simulink model "Template_Simulink_Model_QuanserDCMotor"  (R2018b)
settings: Solver=ode1  StartTime=0.0  StopTime=10  FixedStep=0.001  RelTol=1e-3  EnableMultiTasking=on
undefined symbols (not defined in the file or in its folder): HIL, wf
libraries: quarc_library x3, simulink x1
settings Model: SimulationMode=external  ExtModeTrigDuration=100000  Creator=My Project  LastModifiedBy=Myadmin
settings SolverCC: PositivePriorityOrder=on
settings RTWCC: SystemTargetFile=quarc_linux_rt_armv7.tlc  TemplateMakefile=quarc_linux_rt_armv7_tmf  Description=QUARC Linux RT ARMv7 Target (NI ELVIS III, NI myRIO)
settings STFCustomTargetCC: TargetLibSuffix=.a  TargetPreCompLibLocation=C:\PROGRA~3\QUARC\lib\2018b\LINUX_~1\release  TargetLangStandard=C99 (ISO)  ConcurrentExecutionCompliant=on  GRTInterface=on  SystemTargetFile=quarc_linux_rt_armv7.tlc
settings GRTTargetCC: TargetLibSuffix=.a  TargetPreCompLibLocation=C:\PROGRA~3\QUARC\lib\2018b\LINUX_~1\release  ParMdlRefBuildCompliant=off  CompOptLevelCompliant=off  CombineOutputUpdateFcns=off  MatFileLogging=off  CPPClassGenCompliant=off  GRTInterface=on  UseToolchainInfoCompliant=off  ExtMode=on  ExtModeMexFile=quarc_comm  ExtModeMexArgs='-w -d /tmp -uri %u'

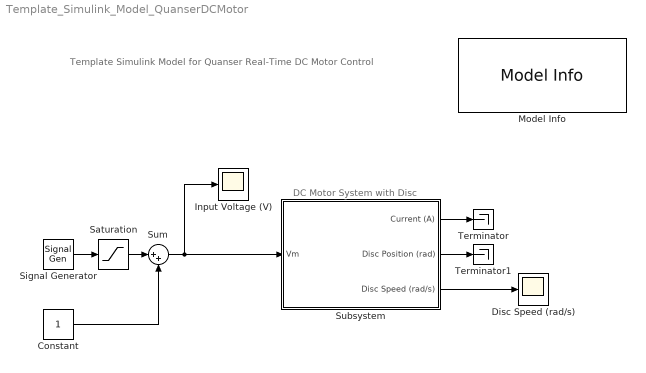
== system Template_Simulink_Model_QuanserDCMotor ==
  note: Template Simulink Model for
      | Quanser Real-Time DC Motor Control
  note: DC Motor System with Disc
  Constant : Constant
  Disc Speed (rad/s) : Scope
  Input Voltage (V) : Scope
  Model Info : simulink/Model-Wide Utilities/Model Info  Frame=off  DisplayStringWithTags=|  HorizontalTextAlignment=Center  LeftAlignmentValue=0.5
      | Model 
      | 
      | %<ModelName>
      | 
      | Dr Arash Khatamianfar
      | EET UNSW 2019
  Saturation : Saturate  UpperLimit=3  LowerLimit=0
  Signal Generator : SignalGenerator  WaveForm=square  Amplitude=2  Frequency=1/4
  Subsystem : Subsystem
  Sum : Sum  Inputs=|++
  Terminator : Terminator
  Terminator1 : Terminator
  wires:
  Constant/1 -> Sum/2
  Signal Generator/1 -> Saturation/1
  Saturation/1 -> Sum/1
  Sum/1 -> Subsystem/1(Vm), Input Voltage (V)/1
  Subsystem/3(Disc Speed (rad/s)) -> Disc Speed (rad/s)/1
  Subsystem/1(Current (A)) -> Terminator/1
  Subsystem/2(Disc Position (rad)) -> Terminator1/1

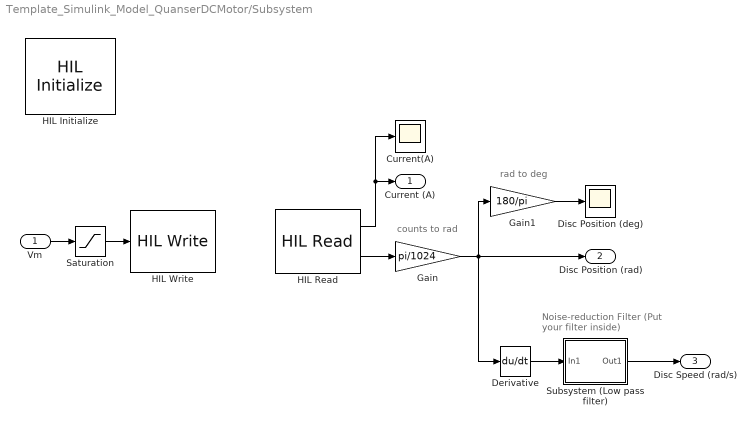
== system Template_Simulink_Model_QuanserDCMotor/Subsystem ==
  note: counts to rad
  note: Noise-reduction Filter
      | (Put your filter inside)
  note: rad to deg
  Vm : Inport
  Current(A) : Scope
  Derivative : Derivative
  Disc Position (deg) : Scope
  Gain : Gain  Gain=pi/1024
  Gain1 : Gain  Gain=180/pi
  HIL Initialize : quarc_library/Data Acquisition/Generic/Configuration/HIL Initialize  object_name=HIL-1  board_type=qab_controls  board_number=0  board_options=""  exclusive=off  active=on  hardware_clocks=[]  clock_modes=[]  initial_clock_frequencies=[]  set_clock_params_at_start=off  set_clock_params_at_switch_in=off  set_clock_frequencies_at_start=off  set_clock_frequencies_at_switch_in=off  analog_input_channels=[0]  analog_input_configurations=[]  analog_input_maximums=[10]  analog_input_minimums=[-10]  set_analog_input_params_at_start=off  set_analog_input_params_at_switch_in=off  analog_output_channels=[0]  analog_output_maximums=[5]  analog_output_minimums=[-5]  initial_analog_outputs=[0]  final_analog_outputs=[0]  watchdog_analog_outputs=[]  set_analog_output_params_at_start=off  set_analog_output_params_at_switch_in=off  set_analog_outputs_at_start=off  set_analog_outputs_at_switch_in=off  set_analog_outputs_at_terminate=on  set_analog_outputs_at_switch_out=off  set_analog_outputs_on_watchdog=off  digital_input_channels=[]  digital_output_channels=[0]  digital_output_configuration=[]  initial_digital_outputs=[1]  final_digital_outputs=[0]  watchdog_digital_outputs=[]  set_digital_output_params_at_start=off  set_digital_output_params_at_switch_in=off  set_digital_outputs_at_start=off  set_digital_outputs_at_switch_in=off  set_digital_outputs_at_terminate=off  set_digital_outputs_at_switch_out=off  set_digital_outputs_on_watchdog=off  encoder_channels=[0:1]  quadrature=[4]  encoder_filter_frequency=[]  initial_encoder_counts=[0]  set_encoder_params_at_start=off  set_encoder_params_at_switch_in=off  set_encoder_counts_at_start=off  set_encoder_counts_at_switch_in=off  pwm_channels=[0]  pwm_modes=0  pwm_frequency=40e6/2047  pwm_configuration=[1]  pwm_alignment=[0]  pwm_polarity=[1]  pwm_leading_deadband=[0]  pwm_trailing_deadband=[0]  initial_pwm_outputs=[0]  final_pwm_outputs=[0]  watchdog_pwm_outputs=[]  set_pwm_params_at_start=off  set_pwm_params_at_switch_in=off  set_pwm_outputs_at_start=off  set_pwm_outputs_at_switch_in=off  set_pwm_outputs_at_terminate=off  set_pwm_outputs_at_switch_out=off  set_pwm_outputs_on_watchdog=off  other_output_channels=[]  initial_other_outputs=[]  final_other_outputs=[]  watchdog_other_outputs=[]  set_other_outputs_at_start=off  set_other_outputs_at_switch_in=off  set_other_outputs_at_terminate=off  set_other_outputs_at_switch_out=off  set_other_outputs_on_watchdog=off
  HIL Read : quarc_library/Data Acquisition/Generic/Immediate I//O/HIL Read  object_name=HIL-1  analog_channels=0  encoder_channels=[0]  digital_channels=[]  other_channels=[]  sample_time=qc_get_step_size  active=on  vector_output=off  data_type_mode=Inherit via back propagation  encoder_data_type=double  digital_data_type=boolean
  HIL Write : quarc_library/Data Acquisition/Generic/Immediate I//O/HIL Write  object_name=HIL-1  analog_channels=0  pwm_channels=[]  digital_channels=[]  other_channels=[]  sample_time=-1  active=off  vector_input=off
  Saturation : Saturate  UpperLimit=5  LowerLimit=-5
  Subsystem (Low pass filter) : Subsystem
  Current (A) : Outport
  Disc Position (rad) : Outport  Port=2
  Disc Speed (rad/s) : Outport  Port=3
  wires:
  Gain/1 -> Disc Position (rad)/1, Gain1/1, Derivative/1
  Subsystem (Low pass filter)/1(Out1) -> Disc Speed (rad/s)/1
  HIL Read/1 -> Current (A)/1, Current(A)/1
  HIL Read/2 -> Gain/1
  Derivative/1 -> Subsystem (Low pass filter)/1(In1)
  Vm/1 -> Saturation/1
  Saturation/1 -> HIL Write/1
  Gain1/1 -> Disc Position (deg)/1

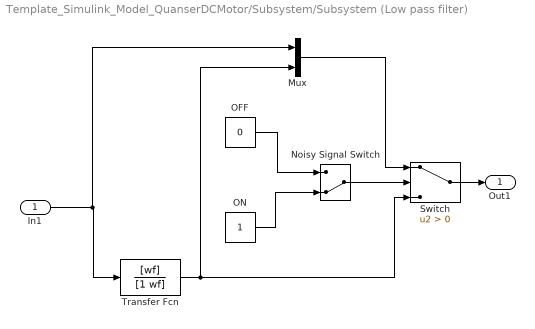
== system Template_Simulink_Model_QuanserDCMotor/Subsystem/Subsystem (Low pass filter) ==
  In1 : Inport
  Mux : Mux  Inputs=2
  Noisy Signal Switch : ManualSwitch  CurrentSetting=0
  OFF : Constant  Value=0
  ON : Constant
  Switch : Switch  Criteria=u2 > Threshold
  Transfer Fcn : TransferFcn  Numerator=[wf]  Denominator=[1 wf]
  Out1 : Outport
  wires:
  In1/1 -> Mux/1, Transfer Fcn/1
  Transfer Fcn/1 -> Mux/2, Switch/3
  Noisy Signal Switch/1 -> Switch/2
  Switch/1 -> Out1/1
  ON/1 -> Noisy Signal Switch/2
  OFF/1 -> Noisy Signal Switch/1
  Mux/1 -> Switch/1
